simulink model "LPVattitudeLQR"  (R2024b)
settings: Solver=ode45  StartTime=0.0  StopTime=tf  RelTol=1e-3
values from neighbouring files (symbols this model uses):
  gamma1_initial = deg2rad(0)    [CMG_Spacecraft_Attitude_Control.m]
  gamma2_initial = deg2rad(90)    [CMG_Spacecraft_Attitude_Control.m]
  p1 = linspace(gamma1_min,gamma1_max,gamma1_points)    [CMG_Spacecraft_Attitude_Control.m]
  p2 = linspace(gamma2_min,gamma2_max,gamma2_points)    [CMG_Spacecraft_Attitude_Control.m]
undefined symbols (not defined in the file or in its folder): K11, K12, K13, K14, K15, K16, K21, K22, K23, K24, K25, K26
libraries: simulink_extras x4, cstblocks x1
settings Model: PacingRate=1000  Creator=lanhi  LastModifiedBy=lanhi

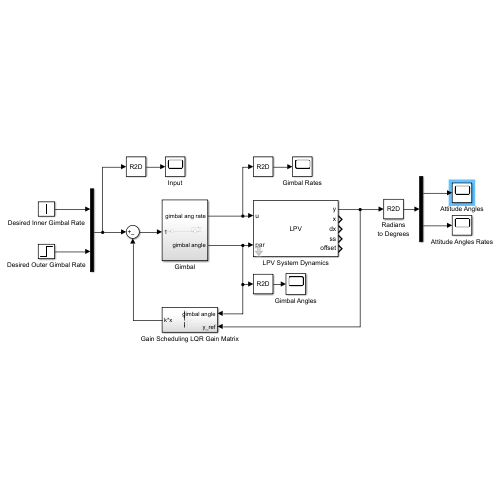
[thumbnail: Simulink's stored preview of the top-level diagram]
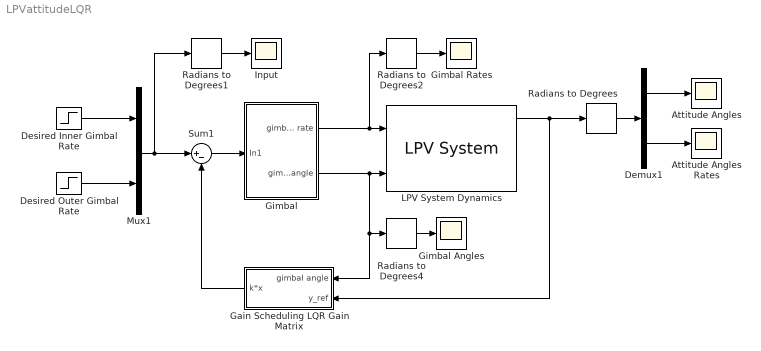
== system LPVattitudeLQR ==
  Attitude Angles : Scope
  Attitude Angles Rates : Scope
  Demux1 : Demux  Outputs=2
  Desired Inner Gimbal Rate : Step  After=0  SampleTime=0
  Desired Outer Gimbal Rate : Step  After=0  SampleTime=0
  Gain Scheduling LQR Gain Matrix : Subsystem
  Gimbal : Subsystem
  Gimbal Angles : Scope
  Gimbal Rates : Scope
  Input : Scope
  LPV System Dynamics : cstblocks/Linear Parameter Varying/LPV System  sys=ICs  InitialConditionSource=internal  InitialCondition=[deg2rad(10) deg2rad(15) deg2rad(-15) deg2rad(-15) deg2rad(5) deg2rad(10)]  opSpecOption=Specify offsets as double arrays  uOffset=0  yOffset=0  xOffset=0  opEquilOption=on  dxOffset=0  AFixed=false  BFixed=false  CFixed=false  DFixed=false  uDelayFixed=false  yDelayFixed=false  iDelayFixed=false  sysFixedOption=First model in state-space array  sysFixed=[]  IMethod=Linear  EMethod=Clip  IndexSearch=Binary search  IndexBegin=on  OutputX=on  OutputXdot=on  OutputLTI=on  OutputOP=on  DataType=double  InitBufferSize=1024  FixedBuffer=off  SimMode=Interpreted execution  Offset=struct
  Mux1 : Mux  Inputs=2
  Radians to Degrees{,1..2,4} (4 alike) : simulink_extras/Transformations/Radians to Degrees
  Sum1 : Sum  Inputs=|+-
  wires:
  Gimbal/2(gimbal angle) -> Gain Scheduling LQR Gain Matrix/1(gimbal angle), Radians to Degrees4/1, LPV System Dynamics/2
  Gain Scheduling LQR Gain Matrix/1(k*x) -> Sum1/2
  LPV System Dynamics/1 -> Radians to Degrees/1, Gain Scheduling LQR Gain Matrix/2(y_ref)
  Desired Inner Gimbal Rate/1 -> Mux1/1
  Desired Outer Gimbal Rate/1 -> Mux1/2
  Demux1/2 -> Attitude Angles Rates/1
  Radians to Degrees4/1 -> Gimbal Angles/1
  Demux1/1 -> Attitude Angles/1
  Radians to Degrees/1 -> Demux1/1
  Sum1/1 -> Gimbal/1(In1)
  Gimbal/1(gimbal ang rate) -> Radians to Degrees2/1, LPV System Dynamics/1
  Radians to Degrees2/1 -> Gimbal Rates/1
  Mux1/1 -> Radians to Degrees1/1, Sum1/1
  Radians to Degrees1/1 -> Input/1

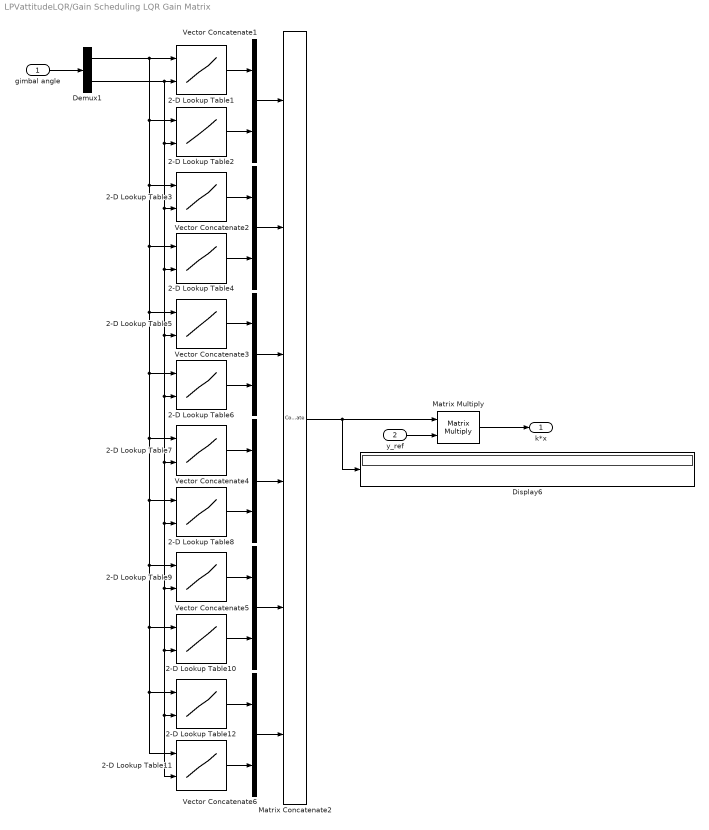
== system LPVattitudeLQR/Gain Scheduling LQR Gain Matrix ==
  gimbal angle : Inport
  y_ref : Inport  Port=2
  2-D Lookup Table1 : Lookup_n-D  BreakpointsForDimension1=p1  BreakpointsForDimension2=p2  Table=K11  InternalRulePriority=Speed  RndMeth=Simplest
      settings: InputPortMap=u0,u1
  2-D Lookup Table10 : Lookup_n-D  BreakpointsForDimension1=p1  BreakpointsForDimension2=p2  Table=K25  InternalRulePriority=Speed  RndMeth=Simplest
      settings: InputPortMap=u0,u1
  2-D Lookup Table11 : Lookup_n-D  BreakpointsForDimension1=p1  BreakpointsForDimension2=p2  Table=K26  InternalRulePriority=Speed  RndMeth=Simplest
      settings: InputPortMap=u0,u1
  2-D Lookup Table12 : Lookup_n-D  BreakpointsForDimension1=p1  BreakpointsForDimension2=p2  Table=K16  InternalRulePriority=Speed  RndMeth=Simplest
      settings: InputPortMap=u0,u1
  2-D Lookup Table2 : Lookup_n-D  BreakpointsForDimension1=p1  BreakpointsForDimension2=p2  Table=K21  InternalRulePriority=Speed  RndMeth=Simplest
      settings: InputPortMap=u0,u1
  2-D Lookup Table3 : Lookup_n-D  BreakpointsForDimension1=p1  BreakpointsForDimension2=p2  Table=K12  InternalRulePriority=Speed  RndMeth=Simplest
      settings: InputPortMap=u0,u1
  2-D Lookup Table4 : Lookup_n-D  BreakpointsForDimension1=p1  BreakpointsForDimension2=p2  Table=K22  InternalRulePriority=Speed  RndMeth=Simplest
      settings: InputPortMap=u0,u1
  2-D Lookup Table5 : Lookup_n-D  BreakpointsForDimension1=p1  BreakpointsForDimension2=p2  Table=K13  InternalRulePriority=Speed  RndMeth=Simplest
      settings: InputPortMap=u0,u1
  2-D Lookup Table6 : Lookup_n-D  BreakpointsForDimension1=p1  BreakpointsForDimension2=p2  Table=K23  InternalRulePriority=Speed  RndMeth=Simplest
      settings: InputPortMap=u0,u1
  2-D Lookup Table7 : Lookup_n-D  BreakpointsForDimension1=p1  BreakpointsForDimension2=p2  Table=K14  InternalRulePriority=Speed  RndMeth=Simplest
      settings: InputPortMap=u0,u1
  2-D Lookup Table8 : Lookup_n-D  BreakpointsForDimension1=p1  BreakpointsForDimension2=p2  Table=K24  InternalRulePriority=Speed  RndMeth=Simplest
      settings: InputPortMap=u0,u1
  2-D Lookup Table9 : Lookup_n-D  BreakpointsForDimension1=p1  BreakpointsForDimension2=p2  Table=K15  InternalRulePriority=Speed  RndMeth=Simplest
      settings: InputPortMap=u0,u1
  Demux1 : Demux  Outputs=2
  Display6 : Display
  Matrix Concatenate2 : Concatenate  NumInputs=6  Mode=Multidimensional array  ConcatenateDimension=2
  Matrix Multiply : Product  Multiplication=Matrix(*)
  Vector Concatenate{1..6} (6 alike) : Concatenate
  k*x : Outport
  wires:
  2-D Lookup Table11/1 -> Vector Concatenate6/2
  Demux1/2 -> 2-D Lookup Table11/2, 2-D Lookup Table12/2, 2-D Lookup Table10/2, 2-D Lookup Table9/2, 2-D Lookup Table8/2, 2-D Lookup Table7/2, 2-D Lookup Table6/2, 2-D Lookup Table5/2, 2-D Lookup Table4/2, 2-D Lookup Table3/2, 2-D Lookup Table2/2, 2-D Lookup Table1/2
  Demux1/1 -> 2-D Lookup Table1/1, 2-D Lookup Table2/1, 2-D Lookup Table3/1, 2-D Lookup Table4/1, 2-D Lookup Table5/1, 2-D Lookup Table6/1, 2-D Lookup Table7/1, 2-D Lookup Table8/1, 2-D Lookup Table9/1, 2-D Lookup Table10/1, 2-D Lookup Table12/1, 2-D Lookup Table11/1
  2-D Lookup Table1/1 -> Vector Concatenate1/1
  2-D Lookup Table2/1 -> Vector Concatenate1/2
  2-D Lookup Table3/1 -> Vector Concatenate2/1
  2-D Lookup Table12/1 -> Vector Concatenate6/1
  2-D Lookup Table5/1 -> Vector Concatenate3/1
  2-D Lookup Table9/1 -> Vector Concatenate5/1
  Vector Concatenate5/1 -> Matrix Concatenate2/5
  2-D Lookup Table7/1 -> Vector Concatenate4/1
  2-D Lookup Table8/1 -> Vector Concatenate4/2
  Vector Concatenate3/1 -> Matrix Concatenate2/3
  2-D Lookup Table10/1 -> Vector Concatenate5/2
  Vector Concatenate6/1 -> Matrix Concatenate2/6
  Vector Concatenate2/1 -> Matrix Concatenate2/2
  Matrix Concatenate2/1 -> Matrix Multiply/1, Display6/1
  Vector Concatenate4/1 -> Matrix Concatenate2/4
  2-D Lookup Table4/1 -> Vector Concatenate2/2
  2-D Lookup Table6/1 -> Vector Concatenate3/2
  Vector Concatenate1/1 -> Matrix Concatenate2/1
  Matrix Multiply/1 -> k*x/1
  gimbal angle/1 -> Demux1/1
  y_ref/1 -> Matrix Multiply/2

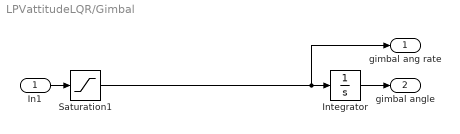
== system LPVattitudeLQR/Gimbal ==
  In1 : Inport
  Integrator : Integrator  InitialCondition=[gamma1_initial,gamma2_initial]
  Saturation1 : Saturate  UpperLimit=9.52  LowerLimit=-9.52
  gimbal ang rate : Outport
  gimbal angle : Outport  Port=2
  wires:
  Integrator/1 -> gimbal angle/1
  In1/1 -> Saturation1/1
  Saturation1/1 -> Integrator/1, gimbal ang rate/1
